simulink model "paperCycle"  (R2020b)
settings: Solver=ode1  StartTime=0.0  StopTime=600  FixedStep=0.002  RelTol=1e-3
values from neighbouring files (symbols this model uses):
  kd = 0.5    [advanced_model_setup.m]    (also in setup_physical.m; simulate_hover.m)
  r = 0.2    [advanced_model_setup.m]    (also in gainScheduling.m = evalin('base', 'r'); setup_physical.m = 2; simulate_hover.m = 0.5)
  skew = 1    [advanced_model_setup.m]    (also in setup_physical.m; simulate_hover.m = 2)
libraries: simulink_extras x2
settings Model: Creator=Jacob  LastModifiedBy=256444
settings DataIOCC: ReturnWorkspaceOutputs=off
settings DebuggingCC: UnconnectedInputMsg=none  UnconnectedOutputMsg=none  UnconnectedLineMsg=none
settings ModelReferenceCC: EnableRefExpFcnMdlSchedulingChecks=off

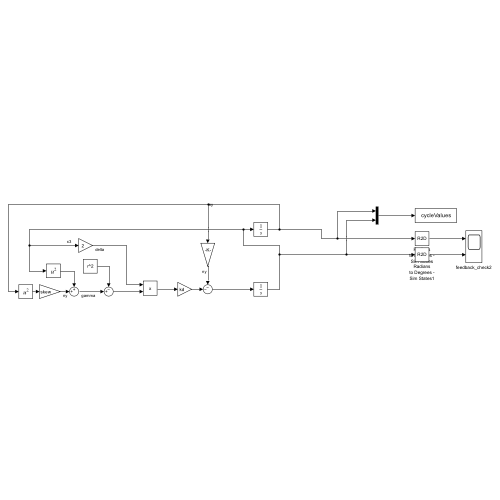
[thumbnail: Simulink's stored preview of the top-level diagram]
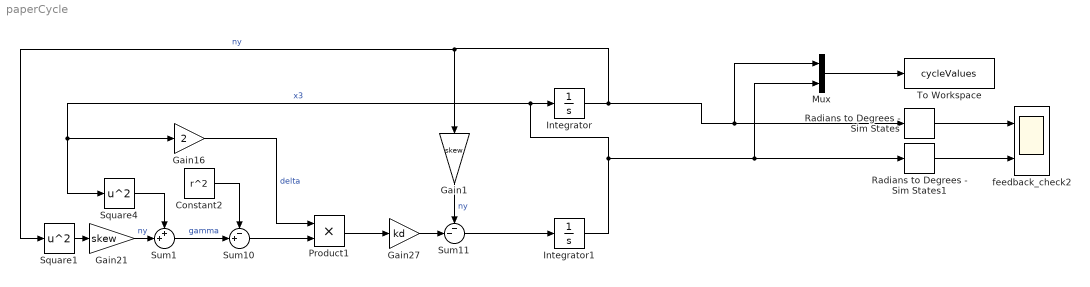
== system paperCycle ==
  Constant2 : Constant  Value=r^2
  Gain1 : Gain  Gain=skew
  Gain16 : Gain  Gain=2
  Gain21 : Gain  Gain=skew
  Gain27 : Gain  Gain=kd
  Integrator : Integrator  InitialCondition=pi/180
  Integrator1 : Integrator  InitialCondition=pi/180
  Mux : Mux  Inputs=2
  Product1 : Product
  Radians to Degrees - Sim States : simulink_extras/Transformations/Radians to Degrees
  Radians to Degrees - Sim States1 : simulink_extras/Transformations/Radians to Degrees
  Square1 : Math  Operator=square  SaturateOnIntegerOverflow=on
  Square4 : Math  Operator=square  SaturateOnIntegerOverflow=on
  Sum1 : Sum  Inputs=++|
  Sum10 : Sum  Inputs=-+|
  Sum11 : Sum  Inputs=--|
  To Workspace : ToWorkspace  VariableName=cycleValues  SampleTime=-1
  feedback_check2 : Scope  NumInputPorts=2
  wires:
  Sum1/1 -> Sum10/2  "gamma"
  Gain21/1 -> Sum1/2  "ny"
  Square4/1 -> Sum1/1
  Square1/1 -> Gain21/1
  Constant2/1 -> Sum10/1
  Gain16/1 -> Product1/1  "delta"
  Integrator1/1 -> Radians to Degrees - Sim States1/1, Mux/2, Square4/1, Gain16/1, Integrator/1  "x3"
  Product1/1 -> Gain27/1
  Sum10/1 -> Product1/2
  Sum11/1 -> Integrator1/1
  Integrator/1 -> Square1/1, Gain1/1, Mux/1, Radians to Degrees - Sim States/1  "ny"
  Gain27/1 -> Sum11/2
  Radians to Degrees - Sim States/1 -> feedback_check2/1
  Radians to Degrees - Sim States1/1 -> feedback_check2/2
  Mux/1 -> To Workspace/1
  Gain1/1 -> Sum11/1  "ny"
